simulink model "gm_max_frequency_index"  (R2020a)
settings: Solver=FixedStepDiscrete  StartTime=0.0  StopTime=1e-2  RelTol=1e-3
model workspace (MAT data in the model file):
  amplitud = 2047
  fft_length = 32
  samples_per_period = 3
  sampling_time = 1e-06
libraries: simulink x384, dspsrcs4 x1, dsphdlxfrm x1, dspstat3 x1, hdlsllib x1
(part 1 of 18)
settings Model: Creator=giova  LastModifiedBy=giova
settings SolverCC: AutoInsertRateTranBlk=on
settings DataIOCC: SaveOutput=off  SaveTime=off
settings OptimizationCC: BlockReduction=off  ConditionallyExecuteInputs=off  DefaultParameterBehavior=Inlined
settings DebuggingCC: AlgebraicLoopMsg=error  InheritedTsInSrcMsg=none  SingleTaskRateTransMsg=error  StrictBusMsg=ErrorOnBusTreatedAsVector  ArithmeticOperatorsInVariantConditions=warning
settings HardwareCC: ProdBitPerPointer=32  ProdBitPerSizeT=32  ProdBitPerPtrDiffT=32  ProdLargestAtomicFloat=None  ProdIntDivRoundTo=Undefined  ProdEndianess=Unspecified  ProdWordSize=32  ProdHWDeviceType=ASIC/FPGA->ASIC/FPGA  TargetBitPerPointer=64  TargetBitPerSizeT=64  TargetBitPerPtrDiffT=64  TargetLongLongMode=on  TargetIntDivRoundTo=Zero  TargetEndianess=LittleEndian  TargetWordSize=64  TargetHWDeviceType=Custom Processor->MATLAB Host Computer  ProdEqTarget=off
settings SFSimCC: SimUseLocalCustomCode=off  CustomCodeUndefinedFunction=UseInterfaceOnly
settings RTWCC: RTWUseLocalCustomCode=off
settings CodeAppCC: StateflowObjectComments=on
settings GRTTargetCC: TargetLangStandard=C89/C90 (ANSI)

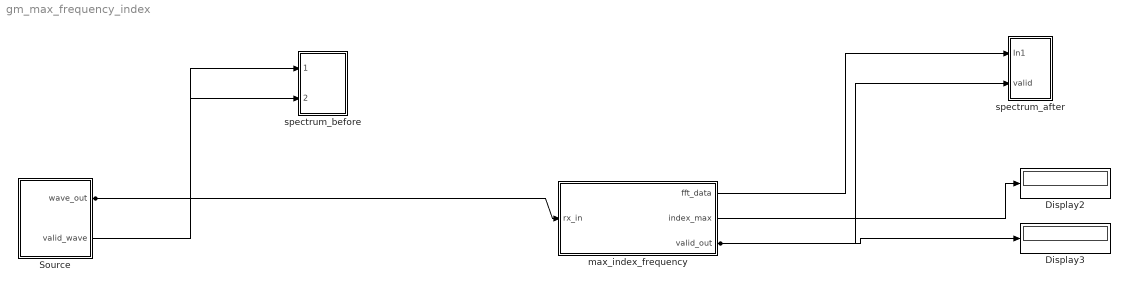
== system gm_max_frequency_index ==
  Display2 : Display
  Display3 : Display
  Source : Subsystem
  max_index_frequency : Subsystem
  spectrum_after : Subsystem
  spectrum_before : Subsystem
  wires:
  max_index_frequency/3(valid_out) -> Display3/1, spectrum_after/2(valid)
  max_index_frequency/2(index_max) -> Display2/1
  max_index_frequency/1(fft_data) -> spectrum_after/1(In1)
  Source/2(valid_wave) -> spectrum_before/2(valid_wave)
  Source/1(wave_out) -> max_index_frequency/1(rx_in), spectrum_before/1(wave_out)

== system gm_max_frequency_index/Source ==
  validated_wave : Subsystem
  wave_out : Outport  VectorParamsAs1DForOutWhenUnconnected=off
  valid_wave : Outport  Port=2  VectorParamsAs1DForOutWhenUnconnected=off
  wires:
  validated_wave/1(wave_out) -> wave_out/1
  validated_wave/2(valid) -> valid_wave/1

== system gm_max_frequency_index/max_index_frequency ==
  rx_in : Inport  OutDataTypeStr=fixdt(1, 12, 0)  PortDimensions=1  SampleTime=1e-06
      settings: SignalType=complex
  FFT_streamer : Subsystem
  frequency_max : Subsystem
  serial2parallel : Subsystem
  fft_data : Outport
  index_max : Outport  Port=2
  valid_out : Outport  Port=3
  wires:
  rx_in/1 -> serial2parallel/1(S)
  FFT_streamer/1(Out1) -> fft_data/1, frequency_max/1(fft_data)
  FFT_streamer/2(Out2) -> frequency_max/2(enable)
  frequency_max/1(index_max) -> index_max/1
  frequency_max/2(valid_out) -> valid_out/1
  serial2parallel/1(P) -> FFT_streamer/1(In1)
  serial2parallel/2(ValidOut) -> FFT_streamer/2(In2)

== system gm_max_frequency_index/spectrum_after ==
  In1 : Inport
  valid : Inport  Port=2
  Abs : Abs  OutDataTypeStr=single
  Cast To Single : DataTypeConversion  OutDataTypeStr=single
  Subsystem : Subsystem
  wires:
  valid/1 -> Subsystem/Enable
  Abs/1 -> Subsystem/1(In1)
  Cast To Single/1 -> Abs/1
  In1/1 -> Cast To Single/1

== system gm_max_frequency_index/spectrum_before ==
  wave_out : Inport
  valid_wave : Inport  Port=2
  Subsystem : Subsystem
  wires:
  valid_wave/1 -> Subsystem/Enable
  wave_out/1 -> Subsystem/1(In1)

== system gm_max_frequency_index/Source/validated_wave ==
  Start_pulse : Subsystem
  Wave_Generator : Subsystem
  wave_out : Outport  VectorParamsAs1DForOutWhenUnconnected=off
  valid : Outport  Port=2  VectorParamsAs1DForOutWhenUnconnected=off
  wires:
  Wave_Generator/1(wave_out) -> wave_out/1
  Start_pulse/1(Out1) -> Wave_Generator/Enable, valid/1

== system gm_max_frequency_index/max_index_frequency/FFT_streamer ==
  In1 : Inport  OutDataTypeStr=fixdt(1, 12, 0)  PortDimensions=[32]  SampleTime=3.2e-05
      settings: SignalType=complex
  In2 : Inport  Port=2  OutDataTypeStr=boolean  PortDimensions=1  SampleTime=3.2e-05
  FFT HDL Optimized : dsphdlxfrm/FFT HDL Optimized  FFTLength=fft_length  Architecture=Streaming Radix 2^2  ComplexMultiplication=Use 3 multipliers and 5 adders  BitReversedOutput=off  BitReversedInput=off  Normalize=on  SimulateUsing=Code generation  RoundingMethod=Floor  ResetInputPort=off  StartOutputPort=off  EndOutputPort=off
      settings: SourceProductBaseCode=DS
  Out1 : Outport
  Out2 : Outport  Port=2
  wires:
  FFT HDL Optimized/1 -> Out1/1
  FFT HDL Optimized/2 -> Out2/1
  In1/1 -> FFT HDL Optimized/1
  In2/1 -> FFT HDL Optimized/2

== system gm_max_frequency_index/max_index_frequency/frequency_max ==
  fft_data : Inport  OutDataTypeStr=fixdt(1, 12, 0)  PortDimensions=[32 1]  SampleTime=3.2e-05
      settings: SignalType=complex
  enable : Inport  Port=2  OutDataTypeStr=boolean  PortDimensions=1  SampleTime=3.2e-05
  index_finder : Subsystem
  index_max : Outport
  valid_out : Outport  Port=2
  wires:
  index_finder/1(index_max) -> index_max/1
  index_finder/2(valid_out) -> valid_out/1
  fft_data/1 -> index_finder/2(fft_data)
  enable/1 -> index_finder/1(enable)

== system gm_max_frequency_index/max_index_frequency/serial2parallel ==
  S : Inport  OutDataTypeStr=fixdt(1, 12, 0)  PortDimensions=1  SampleTime=1e-06
      settings: SignalType=complex
  Deserializer : hdlsllib/HDL Operations/Deserializer1D  Ratio=32  IdleCycles=0  InitialCondition="fi(0,1,12,0,\"hex\",\"000 + 000 i\")"  startIn=off  validIn=off  validOut=on  inputDataDimensions=1  inputSampleTime=1e-06  inputSignalType=complex
      settings: SourceProductBaseCode=SL
  P : Outport
  ValidOut : Outport  Port=2
  wires:
  Deserializer/1 -> P/1
  Deserializer/2 -> ValidOut/1
  S/1 -> Deserializer/1

== system gm_max_frequency_index/spectrum_after/Subsystem ==
  In1 : Inport
  Enable : EnablePort
  Spectrum Analyzer : SpectrumAnalyzer  IsFrequencyInputMode=1
  wires:
  In1/1 -> Spectrum Analyzer/1

== system gm_max_frequency_index/spectrum_before/Subsystem ==
  In1 : Inport
  Enable : EnablePort
  Spectrum Analyzer : SpectrumAnalyzer
  wires:
  In1/1 -> Spectrum Analyzer/1

== system gm_max_frequency_index/Source/validated_wave/Start_pulse ==
  Cast To Boolean : DataTypeConversion  OutDataTypeStr=boolean
  Constant : Constant  SampleTime=sampling_time  LockScale=on
  Out1 : Outport  VectorParamsAs1DForOutWhenUnconnected=off
  wires:
  Constant/1 -> Cast To Boolean/1
  Cast To Boolean/1 -> Out1/1

== system gm_max_frequency_index/Source/validated_wave/Wave_Generator ==
  enable_wave : EnablePort
  complex_wave : dspsrcs4/Sine Wave  Amplitude=amplitud  Frequency=1/(sampling_time*samples_per_period)  Phase=0  SampleMode=Discrete  OutComplex=Complex  CompMethod=Table lookup  TableSize=Speed  SampleTime=sampling_time  SamplesPerFrame=1  ResetState=Restart at time zero  OutputFrames=off  dataType=Fixed-point  wordLen=12  udDataType=sfix(16)  fracBitsMode=User-defined  numFracBits=0  OutDataTypeStr=fixdt(1,12,0)  LastOutDataTypeStr=fixdt(1,12,0)
  wave_out : Outport  InitialOutput=0  VectorParamsAs1DForOutWhenUnconnected=off
  wires:
  complex_wave/1 -> wave_out/1

== system gm_max_frequency_index/max_index_frequency/frequency_max/index_finder ==
  enable : Inport  OutDataTypeStr=boolean  PortDimensions=1  SampleTime=3.2e-05
  fft_data : Inport  Port=2  OutDataTypeStr=fixdt(1, 12, 0)  PortDimensions=[32 1]  SampleTime=3.2e-05
      settings: SignalType=complex
  Data Type Conversion : DataTypeConversion  OutDataTypeStr=uint8  SampleTime=3.2e-05
  Index Vector : MultiPortSwitch  DataPortOrder=Zero-based contiguous  Inputs=1  DiagnosticForDefault=None  zeroidx=on  SampleTime=3.2e-05
  Index Vector_dtc_comp : DataTypeConversion  OutDataTypeStr=fixdt(0, 5, 0)  SampleTime=3.2e-05  RndMeth=Zero
  Maximum : dspstat3/Maximum  operation=maximum  fcn=Index  indexBase=Zero  operateOver=Each column  Dimension=1  InputProcessing=Columns as channels (frame based)  reset=None  roiEnable=off  roiType=Rectangles  roiPortion=Entire ROI  roiOutput=Individual statistics for each ROI  roiFlag=off  roundingMode=Floor  overflowMode=off  prodOutputMode=Binary point scaling  prodOutputWordLength=16  prodOutputFracLength=0  prodOutputDataTypeStr=fixdt([],16,0)  prodOutputLastDataTypeStr=fixdt([],16,0)  accumMode=Binary point scaling  accumWordLength=16  accumFracLength=0  accumDataTypeStr=fixdt([],16,0)  accumLastDataTypeStr=fixdt([],16,0)
  for_each_instance1 : Subsystem
  for_each_instance10 : Subsystem
  for_each_instance11 : Subsystem
  for_each_instance12 : Subsystem
  for_each_instance13 : Subsystem
  for_each_instance14 : Subsystem
  for_each_instance15 : Subsystem
  for_each_instance16 : Subsystem
  for_each_instance17 : Subsystem
  for_each_instance18 : Subsystem
  for_each_instance19 : Subsystem
  for_each_instance2 : Subsystem
  for_each_instance20 : Subsystem
  for_each_instance21 : Subsystem
  for_each_instance22 : Subsystem
  for_each_instance23 : Subsystem
  for_each_instance24 : Subsystem
  for_each_instance25 : Subsystem
  for_each_instance26 : Subsystem
  for_each_instance27 : Subsystem
  for_each_instance28 : Subsystem
  for_each_instance29 : Subsystem
  for_each_instance3 : Subsystem
  for_each_instance30 : Subsystem
  for_each_instance31 : Subsystem
  for_each_instance32 : Subsystem
  for_each_instance4 : Subsystem
  for_each_instance5 : Subsystem
  for_each_instance6 : Subsystem
  for_each_instance7 : Subsystem
  for_each_instance8 : Subsystem
  for_each_instance9 : Subsystem
  t : Concatenate  NumInputs=32
  t1 : Reshape  OutputDimensionality=Column vector (2-D)
  t2 : Concatenate  NumInputs=32
  t3 : Reshape  OutputDimensionality=Column vector (2-D)
  t4 : Demux  Outputs=32
  index_max : Outport
  valid_out : Outport  Port=2
  wires:
  for_each_instance1/1(Out1) -> t2/1
  for_each_instance2/1(Out1) -> t2/2
  for_each_instance3/1(Out1) -> t2/3
  for_each_instance4/1(Out1) -> t2/4
  for_each_instance5/1(Out1) -> t2/5
  for_each_instance6/1(Out1) -> t2/6
  for_each_instance7/1(Out1) -> t2/7
  for_each_instance8/1(Out1) -> t2/8
  for_each_instance9/1(Out1) -> t2/9
  for_each_instance10/1(Out1) -> t2/10
  for_each_instance11/1(Out1) -> t2/11
  for_each_instance12/1(Out1) -> t2/12
  for_each_instance13/1(Out1) -> t2/13
  for_each_instance14/1(Out1) -> t2/14
  for_each_instance15/1(Out1) -> t2/15
  for_each_instance16/1(Out1) -> t2/16
  for_each_instance17/1(Out1) -> t2/17
  for_each_instance18/1(Out1) -> t2/18
  for_each_instance19/1(Out1) -> t2/19
  for_each_instance20/1(Out1) -> t2/20
  for_each_instance21/1(Out1) -> t2/21
  for_each_instance22/1(Out1) -> t2/22
  for_each_instance23/1(Out1) -> t2/23
  for_each_instance24/1(Out1) -> t2/24
  for_each_instance25/1(Out1) -> t2/25
  for_each_instance26/1(Out1) -> t2/26
  for_each_instance27/1(Out1) -> t2/27
  for_each_instance28/1(Out1) -> t2/28
  for_each_instance29/1(Out1) -> t2/29
  for_each_instance30/1(Out1) -> t2/30
  for_each_instance31/1(Out1) -> t2/31
  for_each_instance32/1(Out1) -> t2/32
  for_each_instance1/2(Out2) -> t/1
  for_each_instance2/2(Out2) -> t/2
  for_each_instance3/2(Out2) -> t/3
  for_each_instance4/2(Out2) -> t/4
  for_each_instance5/2(Out2) -> t/5
  for_each_instance6/2(Out2) -> t/6
  for_each_instance7/2(Out2) -> t/7
  for_each_instance8/2(Out2) -> t/8
  for_each_instance9/2(Out2) -> t/9
  for_each_instance10/2(Out2) -> t/10
  for_each_instance11/2(Out2) -> t/11
  for_each_instance12/2(Out2) -> t/12
  for_each_instance13/2(Out2) -> t/13
  for_each_instance14/2(Out2) -> t/14
  for_each_instance15/2(Out2) -> t/15
  for_each_instance16/2(Out2) -> t/16
  for_each_instance17/2(Out2) -> t/17
  for_each_instance18/2(Out2) -> t/18
  for_each_instance19/2(Out2) -> t/19
  for_each_instance20/2(Out2) -> t/20
  for_each_instance21/2(Out2) -> t/21
  for_each_instance22/2(Out2) -> t/22
  for_each_instance23/2(Out2) -> t/23
  for_each_instance24/2(Out2) -> t/24
  for_each_instance25/2(Out2) -> t/25
  for_each_instance26/2(Out2) -> t/26
  for_each_instance27/2(Out2) -> t/27
  for_each_instance28/2(Out2) -> t/28
  for_each_instance29/2(Out2) -> t/29
  for_each_instance30/2(Out2) -> t/30
  for_each_instance31/2(Out2) -> t/31
  for_each_instance32/2(Out2) -> t/32
  Data Type Conversion/1 -> index_max/1
  Index Vector/1 -> valid_out/1
  t4/1 -> for_each_instance1/1(fft_data)
  t4/2 -> for_each_instance2/1(fft_data)
  t4/3 -> for_each_instance3/1(fft_data)
  t4/4 -> for_each_instance4/1(fft_data)
  t4/5 -> for_each_instance5/1(fft_data)
  t4/6 -> for_each_instance6/1(fft_data)
  t4/7 -> for_each_instance7/1(fft_data)
  t4/8 -> for_each_instance8/1(fft_data)
  t4/9 -> for_each_instance9/1(fft_data)
  t4/10 -> for_each_instance10/1(fft_data)
  t4/11 -> for_each_instance11/1(fft_data)
  t4/12 -> for_each_instance12/1(fft_data)
  t4/13 -> for_each_instance13/1(fft_data)
  t4/14 -> for_each_instance14/1(fft_data)
  t4/15 -> for_each_instance15/1(fft_data)
  t4/16 -> for_each_instance16/1(fft_data)
  t4/17 -> for_each_instance17/1(fft_data)
  t4/18 -> for_each_instance18/1(fft_data)
  t4/19 -> for_each_instance19/1(fft_data)
  t4/20 -> for_each_instance20/1(fft_data)
  t4/21 -> for_each_instance21/1(fft_data)
  t4/22 -> for_each_instance22/1(fft_data)
  t4/23 -> for_each_instance23/1(fft_data)
  t4/24 -> for_each_instance24/1(fft_data)
  t4/25 -> for_each_instance25/1(fft_data)
  t4/26 -> for_each_instance26/1(fft_data)
  t4/27 -> for_each_instance27/1(fft_data)
  t4/28 -> for_each_instance28/1(fft_data)
  t4/29 -> for_each_instance29/1(fft_data)
  t4/30 -> for_each_instance30/1(fft_data)
  t4/31 -> for_each_instance31/1(fft_data)
  t4/32 -> for_each_instance32/1(fft_data)
  enable/1 -> for_each_instance32/2(enable), for_each_instance31/2(enable), for_each_instance30/2(enable), for_each_instance29/2(enable), for_each_instance28/2(enable), for_each_instance27/2(enable), for_each_instance26/2(enable), for_each_instance25/2(enable), for_each_instance24/2(enable), for_each_instance23/2(enable), for_each_instance22/2(enable), for_each_instance21/2(enable), for_each_instance20/2(enable), for_each_instance19/2(enable), for_each_instance18/2(enable), for_each_instance17/2(enable), for_each_instance16/2(enable), for_each_instance15/2(enable), for_each_instance14/2(enable), for_each_instance13/2(enable), for_each_instance12/2(enable), for_each_instance11/2(enable), for_each_instance10/2(enable), for_each_instance9/2(enable), for_each_instance8/2(enable), for_each_instance7/2(enable), for_each_instance6/2(enable), for_each_instance5/2(enable), for_each_instance4/2(enable), for_each_instance3/2(enable), for_each_instance2/2(enable), for_each_instance1/2(enable)
  fft_data/1 -> t4/1
  t/1 -> t1/1
  t1/1 -> Index Vector/2
  t2/1 -> t3/1
  t3/1 -> Maximum/1
  Maximum/1 -> Data Type Conversion/1, Index Vector_dtc_comp/1
  Index Vector_dtc_comp/1 -> Index Vector/1

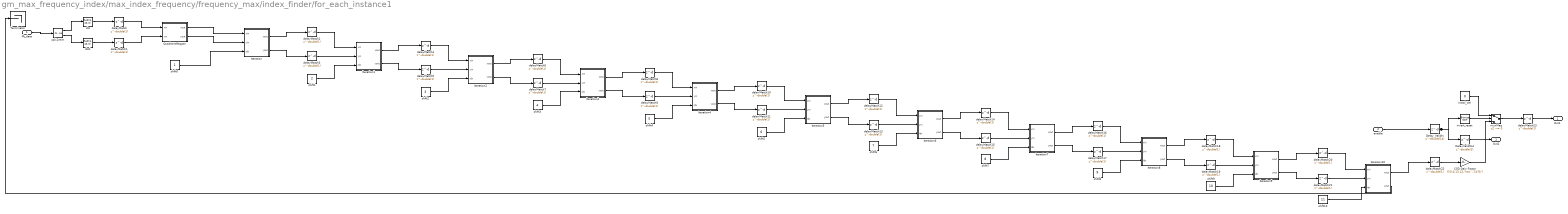
== system gm_max_frequency_index/max_index_frequency/frequency_max/index_finder/for_each_instance1 ==
  fft_data : Inport  OutDataTypeStr=fixdt(1, 12, 0)  PortDimensions=1  SampleTime=3.2e-05
      settings: SignalType=complex
  enable : Inport  Port=2  OutDataTypeStr=boolean  PortDimensions=1  SampleTime=3.2e-05
  CSD Gain Factor : Gain  Gain="fi(0,0,13,13,\"hex\",\"1b7b\")"  ParamDataTypeStr=fixdt(0, 13, 13)  OutDataTypeStr=fixdt(1, 13, 0)  SampleTime=3.2e-05
  DelayValidOut : Delay  DelayLength=double(1)  InitialCondition=0  SampleTime=3.2e-05
  Delay_ValidIn : Delay  DelayLength=double(14)  InitialCondition=0  SampleTime=3.2e-05
  Initial_Val : Constant  Value=0  OutDataTypeStr=fixdt(1, 13, 0)  SampleTime=3.2e-05
  Iteration : Subsystem
  Iteration1 : Subsystem
  Iteration10 : Subsystem
  Iteration2 : Subsystem
  Iteration3 : Subsystem
  Iteration4 : Subsystem
  Iteration5 : Subsystem
  Iteration6 : Subsystem
  Iteration7 : Subsystem
  Iteration8 : Subsystem
  Iteration9 : Subsystem
  QuadrantMapper : Subsystem
  Terminator : Terminator
  cplx2reim : ComplexToRealImag  SampleTime=3.2e-05
  delayMatch{,1..23} (24 alike) : Delay  DelayLength=double(1)  InitialCondition=0  SampleTime=3.2e-05
  dtc : DataTypeConversion  OutDataTypeStr=fixdt(1, 13, 0)  SampleTime=3.2e-05
  dtc1 : DataTypeConversion  OutDataTypeStr=fixdt(1, 13, 0)  SampleTime=3.2e-05
  invert_reset : simulink/Logic and Bit Operations/Bitwise Operator  logicop=NOT  UseBitMask=off  BitMask=double(0)  BitMaskRealWorld=Real World Value
  muxMag : Switch  Criteria=u2 ~= 0  Threshold=double(0)  OutDataTypeStr=fixdt(1, 13, 0)  SampleTime=3.2e-05
  shift0 : Constant  VectorParams1D=off  OutDataTypeStr=fixdt(0, 5, 0)  SampleTime=3.2e-05
  shift1 : Constant  Value=2  VectorParams1D=off  OutDataTypeStr=fixdt(0, 5, 0)  SampleTime=3.2e-05
  shift10 : Constant  Value=11  VectorParams1D=off  OutDataTypeStr=fixdt(0, 5, 0)  SampleTime=3.2e-05
  shift2 : Constant  Value=3  VectorParams1D=off  OutDataTypeStr=fixdt(0, 5, 0)  SampleTime=3.2e-05
  shift3 : Constant  Value=4  VectorParams1D=off  OutDataTypeStr=fixdt(0, 5, 0)  SampleTime=3.2e-05
  shift4 : Constant  Value=5  VectorParams1D=off  OutDataTypeStr=fixdt(0, 5, 0)  SampleTime=3.2e-05
  shift5 : Constant  Value=6  VectorParams1D=off  OutDataTypeStr=fixdt(0, 5, 0)  SampleTime=3.2e-05
  shift6 : Constant  Value=7  VectorParams1D=off  OutDataTypeStr=fixdt(0, 5, 0)  SampleTime=3.2e-05
  shift7 : Constant  Value=8  VectorParams1D=off  OutDataTypeStr=fixdt(0, 5, 0)  SampleTime=3.2e-05
  shift8 : Constant  Value=9  VectorParams1D=off  OutDataTypeStr=fixdt(0, 5, 0)  SampleTime=3.2e-05
  shift9 : Constant  Value=10  VectorParams1D=off  OutDataTypeStr=fixdt(0, 5, 0)  SampleTime=3.2e-05
  Out1 : Outport
  Out2 : Outport  Port=2  VectorParamsAs1DForOutWhenUnconnected=off
  wires:
  DelayValidOut/1 -> Out2/1
  delayMatch2/1 -> Iteration1/1(xin)
  delayMatch3/1 -> Iteration1/2(yin)
  delayMatch4/1 -> Iteration2/1(xin)
  delayMatch5/1 -> Iteration2/2(yin)
  delayMatch6/1 -> Iteration3/1(xin)
  delayMatch7/1 -> Iteration3/2(yin)
  delayMatch8/1 -> Iteration4/1(xin)
  delayMatch9/1 -> Iteration4/2(yin)
  delayMatch10/1 -> Iteration5/1(xin)
  delayMatch11/1 -> Iteration5/2(yin)
  delayMatch12/1 -> Iteration6/1(xin)
  delayMatch13/1 -> Iteration6/2(yin)
  delayMatch14/1 -> Iteration7/1(xin)
  delayMatch15/1 -> Iteration7/2(yin)
  delayMatch16/1 -> Iteration8/1(xin)
  delayMatch17/1 -> Iteration8/2(yin)
  delayMatch18/1 -> Iteration9/1(xin)
  delayMatch19/1 -> Iteration9/2(yin)
  delayMatch20/1 -> Iteration10/1(xin)
  delayMatch21/1 -> Iteration10/2(yin)
  delayMatch22/1 -> CSD Gain Factor/1
  delayMatch/1 -> QuadrantMapper/1(xin)
  delayMatch1/1 -> QuadrantMapper/2(yin)
  QuadrantMapper/1(xout) -> Iteration/1(xin)
  QuadrantMapper/2(yout) -> Iteration/2(yin)
  Delay_ValidIn/1 -> DelayValidOut/1, invert_reset/1
  delayMatch23/1 -> Out1/1
  fft_data/1 -> cplx2reim/1
  enable/1 -> Delay_ValidIn/1
  cplx2reim/1 -> dtc/1
  cplx2reim/2 -> dtc1/1
  dtc/1 -> delayMatch/1
  dtc1/1 -> delayMatch1/1
  shift0/1 -> Iteration/3(idx)
  Iteration/1(xout) -> delayMatch2/1
  Iteration/2(yout) -> delayMatch3/1
  shift1/1 -> Iteration1/3(idx)
  Iteration1/1(xout) -> delayMatch4/1
  Iteration1/2(yout) -> delayMatch5/1
  shift2/1 -> Iteration2/3(idx)
  Iteration2/1(xout) -> delayMatch6/1
  Iteration2/2(yout) -> delayMatch7/1
  shift3/1 -> Iteration3/3(idx)
  Iteration3/1(xout) -> delayMatch8/1
  Iteration3/2(yout) -> delayMatch9/1
  shift4/1 -> Iteration4/3(idx)
  Iteration4/1(xout) -> delayMatch10/1
  Iteration4/2(yout) -> delayMatch11/1
  shift5/1 -> Iteration5/3(idx)
  Iteration5/1(xout) -> delayMatch12/1
  Iteration5/2(yout) -> delayMatch13/1
  shift6/1 -> Iteration6/3(idx)
  Iteration6/1(xout) -> delayMatch14/1
  Iteration6/2(yout) -> delayMatch15/1
  shift7/1 -> Iteration7/3(idx)
  Iteration7/1(xout) -> delayMatch16/1
  Iteration7/2(yout) -> delayMatch17/1
  shift8/1 -> Iteration8/3(idx)
  Iteration8/1(xout) -> delayMatch18/1
  Iteration8/2(yout) -> delayMatch19/1
  shift9/1 -> Iteration9/3(idx)
  Iteration9/1(xout) -> delayMatch20/1
  Iteration9/2(yout) -> delayMatch21/1
  Iteration10/2(yout) -> Terminator/1
  shift10/1 -> Iteration10/3(idx)
  Iteration10/1(xout) -> delayMatch22/1
  Initial_Val/1 -> muxMag/1
  CSD Gain Factor/1 -> muxMag/3
  invert_reset/1 -> muxMag/2
  muxMag/1 -> delayMatch23/1

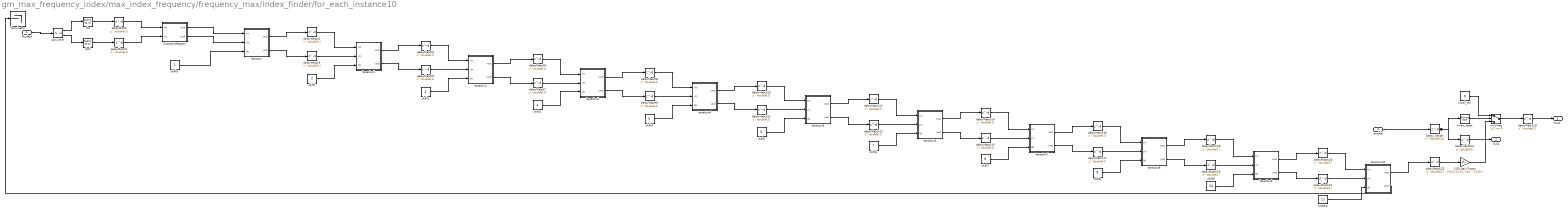
== system gm_max_frequency_index/max_index_frequency/frequency_max/index_finder/for_each_instance10 ==
  fft_data : Inport  OutDataTypeStr=fixdt(1, 12, 0)  PortDimensions=1  SampleTime=3.2e-05
      settings: SignalType=complex
  enable : Inport  Port=2  OutDataTypeStr=boolean  PortDimensions=1  SampleTime=3.2e-05
  CSD Gain Factor : Gain  Gain="fi(0,0,13,13,\"hex\",\"1b7b\")"  ParamDataTypeStr=fixdt(0, 13, 13)  OutDataTypeStr=fixdt(1, 13, 0)  SampleTime=3.2e-05
  DelayValidOut : Delay  DelayLength=double(1)  InitialCondition=0  SampleTime=3.2e-05
  Delay_ValidIn : Delay  DelayLength=double(14)  InitialCondition=0  SampleTime=3.2e-05
  Initial_Val : Constant  Value=0  OutDataTypeStr=fixdt(1, 13, 0)  SampleTime=3.2e-05
  Iteration : Subsystem
  Iteration1 : Subsystem
  Iteration10 : Subsystem
  Iteration2 : Subsystem
  Iteration3 : Subsystem
  Iteration4 : Subsystem
  Iteration5 : Subsystem
  Iteration6 : Subsystem
  Iteration7 : Subsystem
  Iteration8 : Subsystem
  Iteration9 : Subsystem
  QuadrantMapper : Subsystem
  Terminator : Terminator
  cplx2reim : ComplexToRealImag  SampleTime=3.2e-05
  delayMatch{,1..23} (24 alike) : Delay  DelayLength=double(1)  InitialCondition=0  SampleTime=3.2e-05
  dtc : DataTypeConversion  OutDataTypeStr=fixdt(1, 13, 0)  SampleTime=3.2e-05
  dtc1 : DataTypeConversion  OutDataTypeStr=fixdt(1, 13, 0)  SampleTime=3.2e-05
  invert_reset : simulink/Logic and Bit Operations/Bitwise Operator  logicop=NOT  UseBitMask=off  BitMask=double(0)  BitMaskRealWorld=Real World Value
  muxMag : Switch  Criteria=u2 ~= 0  Threshold=double(0)  OutDataTypeStr=fixdt(1, 13, 0)  SampleTime=3.2e-05
  shift0 : Constant  VectorParams1D=off  OutDataTypeStr=fixdt(0, 5, 0)  SampleTime=3.2e-05
  shift1 : Constant  Value=2  VectorParams1D=off  OutDataTypeStr=fixdt(0, 5, 0)  SampleTime=3.2e-05
  shift10 : Constant  Value=11  VectorParams1D=off  OutDataTypeStr=fixdt(0, 5, 0)  SampleTime=3.2e-05
  shift2 : Constant  Value=3  VectorParams1D=off  OutDataTypeStr=fixdt(0, 5, 0)  SampleTime=3.2e-05
  shift3 : Constant  Value=4  VectorParams1D=off  OutDataTypeStr=fixdt(0, 5, 0)  SampleTime=3.2e-05
  shift4 : Constant  Value=5  VectorParams1D=off  OutDataTypeStr=fixdt(0, 5, 0)  SampleTime=3.2e-05
  shift5 : Constant  Value=6  VectorParams1D=off  OutDataTypeStr=fixdt(0, 5, 0)  SampleTime=3.2e-05
  shift6 : Constant  Value=7  VectorParams1D=off  OutDataTypeStr=fixdt(0, 5, 0)  SampleTime=3.2e-05
  shift7 : Constant  Value=8  VectorParams1D=off  OutDataTypeStr=fixdt(0, 5, 0)  SampleTime=3.2e-05
  shift8 : Constant  Value=9  VectorParams1D=off  OutDataTypeStr=fixdt(0, 5, 0)  SampleTime=3.2e-05
  shift9 : Constant  Value=10  VectorParams1D=off  OutDataTypeStr=fixdt(0, 5, 0)  SampleTime=3.2e-05
  Out1 : Outport
  Out2 : Outport  Port=2  VectorParamsAs1DForOutWhenUnconnected=off
  wires:
  muxMag/1 -> delayMatch23/1
  invert_reset/1 -> muxMag/2
  CSD Gain Factor/1 -> muxMag/3
  Initial_Val/1 -> muxMag/1
  Iteration10/1(xout) -> delayMatch22/1
  shift10/1 -> Iteration10/3(idx)
  Iteration10/2(yout) -> Terminator/1
  Iteration9/2(yout) -> delayMatch21/1
  Iteration9/1(xout) -> delayMatch20/1
  shift9/1 -> Iteration9/3(idx)
  Iteration8/2(yout) -> delayMatch19/1
  Iteration8/1(xout) -> delayMatch18/1
  shift8/1 -> Iteration8/3(idx)
  Iteration7/2(yout) -> delayMatch17/1
  Iteration7/1(xout) -> delayMatch16/1
  shift7/1 -> Iteration7/3(idx)
  Iteration6/2(yout) -> delayMatch15/1
  Iteration6/1(xout) -> delayMatch14/1
  shift6/1 -> Iteration6/3(idx)
  Iteration5/2(yout) -> delayMatch13/1
  Iteration5/1(xout) -> delayMatch12/1
  shift5/1 -> Iteration5/3(idx)
  Iteration4/2(yout) -> delayMatch11/1
  Iteration4/1(xout) -> delayMatch10/1
  shift4/1 -> Iteration4/3(idx)
  Iteration3/2(yout) -> delayMatch9/1
  Iteration3/1(xout) -> delayMatch8/1
  shift3/1 -> Iteration3/3(idx)
  Iteration2/2(yout) -> delayMatch7/1
  Iteration2/1(xout) -> delayMatch6/1
  shift2/1 -> Iteration2/3(idx)
  Iteration1/2(yout) -> delayMatch5/1
  Iteration1/1(xout) -> delayMatch4/1
  shift1/1 -> Iteration1/3(idx)
  Iteration/2(yout) -> delayMatch3/1
  Iteration/1(xout) -> delayMatch2/1
  shift0/1 -> Iteration/3(idx)
  dtc1/1 -> delayMatch1/1
  dtc/1 -> delayMatch/1
  cplx2reim/2 -> dtc1/1
  cplx2reim/1 -> dtc/1
  enable/1 -> Delay_ValidIn/1
  fft_data/1 -> cplx2reim/1
  delayMatch23/1 -> Out1/1
  Delay_ValidIn/1 -> invert_reset/1, DelayValidOut/1
  QuadrantMapper/2(yout) -> Iteration/2(yin)
  QuadrantMapper/1(xout) -> Iteration/1(xin)
  delayMatch1/1 -> QuadrantMapper/2(yin)
  delayMatch/1 -> QuadrantMapper/1(xin)
  delayMatch22/1 -> CSD Gain Factor/1
  delayMatch21/1 -> Iteration10/2(yin)
  delayMatch20/1 -> Iteration10/1(xin)
  delayMatch19/1 -> Iteration9/2(yin)
  delayMatch18/1 -> Iteration9/1(xin)
  delayMatch17/1 -> Iteration8/2(yin)
  delayMatch16/1 -> Iteration8/1(xin)
  delayMatch15/1 -> Iteration7/2(yin)
  delayMatch14/1 -> Iteration7/1(xin)
  delayMatch13/1 -> Iteration6/2(yin)
  delayMatch12/1 -> Iteration6/1(xin)
  delayMatch11/1 -> Iteration5/2(yin)
  delayMatch10/1 -> Iteration5/1(xin)
  delayMatch9/1 -> Iteration4/2(yin)
  delayMatch8/1 -> Iteration4/1(xin)
  delayMatch7/1 -> Iteration3/2(yin)
  delayMatch6/1 -> Iteration3/1(xin)
  delayMatch5/1 -> Iteration2/2(yin)
  delayMatch4/1 -> Iteration2/1(xin)
  delayMatch3/1 -> Iteration1/2(yin)
  delayMatch2/1 -> Iteration1/1(xin)
  DelayValidOut/1 -> Out2/1

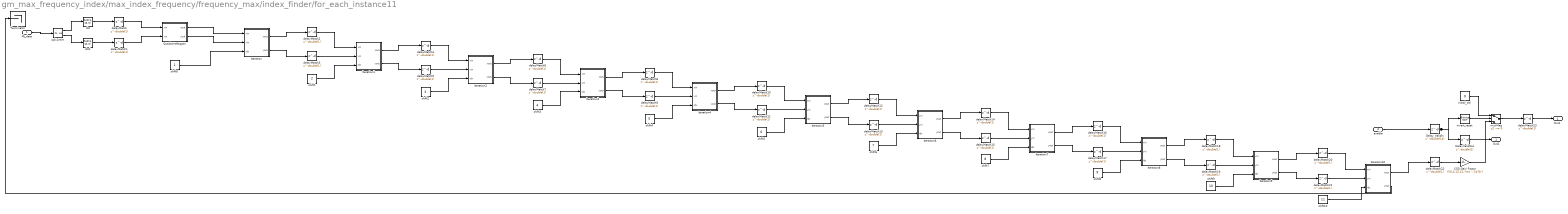
== system gm_max_frequency_index/max_index_frequency/frequency_max/index_finder/for_each_instance11 ==
  fft_data : Inport  OutDataTypeStr=fixdt(1, 12, 0)  PortDimensions=1  SampleTime=3.2e-05
      settings: SignalType=complex
  enable : Inport  Port=2  OutDataTypeStr=boolean  PortDimensions=1  SampleTime=3.2e-05
  CSD Gain Factor : Gain  Gain="fi(0,0,13,13,\"hex\",\"1b7b\")"  ParamDataTypeStr=fixdt(0, 13, 13)  OutDataTypeStr=fixdt(1, 13, 0)  SampleTime=3.2e-05
  DelayValidOut : Delay  DelayLength=double(1)  InitialCondition=0  SampleTime=3.2e-05
  Delay_ValidIn : Delay  DelayLength=double(14)  InitialCondition=0  SampleTime=3.2e-05
  Initial_Val : Constant  Value=0  OutDataTypeStr=fixdt(1, 13, 0)  SampleTime=3.2e-05
  Iteration : Subsystem
  Iteration1 : Subsystem
  Iteration10 : Subsystem
  Iteration2 : Subsystem
  Iteration3 : Subsystem
  Iteration4 : Subsystem
  Iteration5 : Subsystem
  Iteration6 : Subsystem
  Iteration7 : Subsystem
  Iteration8 : Subsystem
  Iteration9 : Subsystem
  QuadrantMapper : Subsystem
  Terminator : Terminator
  cplx2reim : ComplexToRealImag  SampleTime=3.2e-05
  delayMatch{,1..23} (24 alike) : Delay  DelayLength=double(1)  InitialCondition=0  SampleTime=3.2e-05
  dtc : DataTypeConversion  OutDataTypeStr=fixdt(1, 13, 0)  SampleTime=3.2e-05
  dtc1 : DataTypeConversion  OutDataTypeStr=fixdt(1, 13, 0)  SampleTime=3.2e-05
  invert_reset : simulink/Logic and Bit Operations/Bitwise Operator  logicop=NOT  UseBitMask=off  BitMask=double(0)  BitMaskRealWorld=Real World Value
  muxMag : Switch  Criteria=u2 ~= 0  Threshold=double(0)  OutDataTypeStr=fixdt(1, 13, 0)  SampleTime=3.2e-05
  shift0 : Constant  VectorParams1D=off  OutDataTypeStr=fixdt(0, 5, 0)  SampleTime=3.2e-05
  shift1 : Constant  Value=2  VectorParams1D=off  OutDataTypeStr=fixdt(0, 5, 0)  SampleTime=3.2e-05
  shift10 : Constant  Value=11  VectorParams1D=off  OutDataTypeStr=fixdt(0, 5, 0)  SampleTime=3.2e-05
  shift2 : Constant  Value=3  VectorParams1D=off  OutDataTypeStr=fixdt(0, 5, 0)  SampleTime=3.2e-05
  shift3 : Constant  Value=4  VectorParams1D=off  OutDataTypeStr=fixdt(0, 5, 0)  SampleTime=3.2e-05
  shift4 : Constant  Value=5  VectorParams1D=off  OutDataTypeStr=fixdt(0, 5, 0)  SampleTime=3.2e-05
  shift5 : Constant  Value=6  VectorParams1D=off  OutDataTypeStr=fixdt(0, 5, 0)  SampleTime=3.2e-05
  shift6 : Constant  Value=7  VectorParams1D=off  OutDataTypeStr=fixdt(0, 5, 0)  SampleTime=3.2e-05
  shift7 : Constant  Value=8  VectorParams1D=off  OutDataTypeStr=fixdt(0, 5, 0)  SampleTime=3.2e-05
  shift8 : Constant  Value=9  VectorParams1D=off  OutDataTypeStr=fixdt(0, 5, 0)  SampleTime=3.2e-05
  shift9 : Constant  Value=10  VectorParams1D=off  OutDataTypeStr=fixdt(0, 5, 0)  SampleTime=3.2e-05
  Out1 : Outport
  Out2 : Outport  Port=2  VectorParamsAs1DForOutWhenUnconnected=off
  wires:
  muxMag/1 -> delayMatch23/1
  invert_reset/1 -> muxMag/2
  CSD Gain Factor/1 -> muxMag/3
  Initial_Val/1 -> muxMag/1
  Iteration10/1(xout) -> delayMatch22/1
  shift10/1 -> Iteration10/3(idx)
  Iteration10/2(yout) -> Terminator/1
  Iteration9/2(yout) -> delayMatch21/1
  Iteration9/1(xout) -> delayMatch20/1
  shift9/1 -> Iteration9/3(idx)
  Iteration8/2(yout) -> delayMatch19/1
  Iteration8/1(xout) -> delayMatch18/1
  shift8/1 -> Iteration8/3(idx)
  Iteration7/2(yout) -> delayMatch17/1
  Iteration7/1(xout) -> delayMatch16/1
  shift7/1 -> Iteration7/3(idx)
  Iteration6/2(yout) -> delayMatch15/1
  Iteration6/1(xout) -> delayMatch14/1
  shift6/1 -> Iteration6/3(idx)
  Iteration5/2(yout) -> delayMatch13/1
  Iteration5/1(xout) -> delayMatch12/1
  shift5/1 -> Iteration5/3(idx)
  Iteration4/2(yout) -> delayMatch11/1
  Iteration4/1(xout) -> delayMatch10/1
  shift4/1 -> Iteration4/3(idx)
  Iteration3/2(yout) -> delayMatch9/1
  Iteration3/1(xout) -> delayMatch8/1
  shift3/1 -> Iteration3/3(idx)
  Iteration2/2(yout) -> delayMatch7/1
  Iteration2/1(xout) -> delayMatch6/1
  shift2/1 -> Iteration2/3(idx)
  Iteration1/2(yout) -> delayMatch5/1
  Iteration1/1(xout) -> delayMatch4/1
  shift1/1 -> Iteration1/3(idx)
  Iteration/2(yout) -> delayMatch3/1
  Iteration/1(xout) -> delayMatch2/1
  shift0/1 -> Iteration/3(idx)
  dtc1/1 -> delayMatch1/1
  dtc/1 -> delayMatch/1
  cplx2reim/2 -> dtc1/1
  cplx2reim/1 -> dtc/1
  enable/1 -> Delay_ValidIn/1
  fft_data/1 -> cplx2reim/1
  delayMatch23/1 -> Out1/1
  Delay_ValidIn/1 -> invert_reset/1, DelayValidOut/1
  QuadrantMapper/2(yout) -> Iteration/2(yin)
  QuadrantMapper/1(xout) -> Iteration/1(xin)
  delayMatch1/1 -> QuadrantMapper/2(yin)
  delayMatch/1 -> QuadrantMapper/1(xin)
  delayMatch22/1 -> CSD Gain Factor/1
  delayMatch21/1 -> Iteration10/2(yin)
  delayMatch20/1 -> Iteration10/1(xin)
  delayMatch19/1 -> Iteration9/2(yin)
  delayMatch18/1 -> Iteration9/1(xin)
  delayMatch17/1 -> Iteration8/2(yin)
  delayMatch16/1 -> Iteration8/1(xin)
  delayMatch15/1 -> Iteration7/2(yin)
  delayMatch14/1 -> Iteration7/1(xin)
  delayMatch13/1 -> Iteration6/2(yin)
  delayMatch12/1 -> Iteration6/1(xin)
  delayMatch11/1 -> Iteration5/2(yin)
  delayMatch10/1 -> Iteration5/1(xin)
  delayMatch9/1 -> Iteration4/2(yin)
  delayMatch8/1 -> Iteration4/1(xin)
  delayMatch7/1 -> Iteration3/2(yin)
  delayMatch6/1 -> Iteration3/1(xin)
  delayMatch5/1 -> Iteration2/2(yin)
  delayMatch4/1 -> Iteration2/1(xin)
  delayMatch3/1 -> Iteration1/2(yin)
  delayMatch2/1 -> Iteration1/1(xin)
  DelayValidOut/1 -> Out2/1

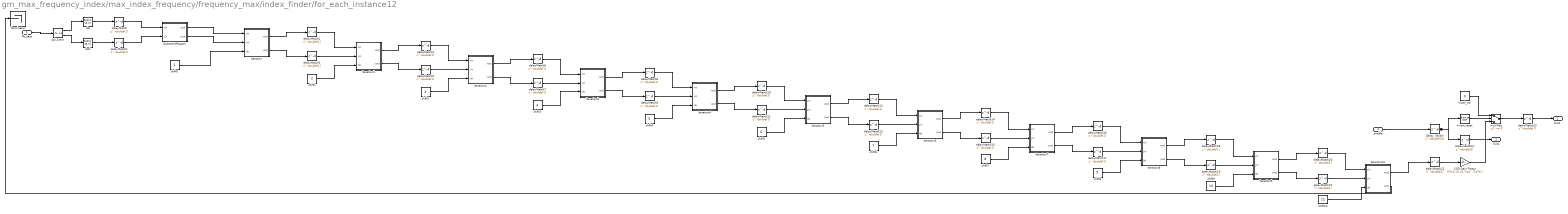
== system gm_max_frequency_index/max_index_frequency/frequency_max/index_finder/for_each_instance12 ==
  fft_data : Inport  OutDataTypeStr=fixdt(1, 12, 0)  PortDimensions=1  SampleTime=3.2e-05
      settings: SignalType=complex
  enable : Inport  Port=2  OutDataTypeStr=boolean  PortDimensions=1  SampleTime=3.2e-05
  CSD Gain Factor : Gain  Gain="fi(0,0,13,13,\"hex\",\"1b7b\")"  ParamDataTypeStr=fixdt(0, 13, 13)  OutDataTypeStr=fixdt(1, 13, 0)  SampleTime=3.2e-05
  DelayValidOut : Delay  DelayLength=double(1)  InitialCondition=0  SampleTime=3.2e-05
  Delay_ValidIn : Delay  DelayLength=double(14)  InitialCondition=0  SampleTime=3.2e-05
  Initial_Val : Constant  Value=0  OutDataTypeStr=fixdt(1, 13, 0)  SampleTime=3.2e-05
  Iteration : Subsystem
  Iteration1 : Subsystem
  Iteration10 : Subsystem
  Iteration2 : Subsystem
  Iteration3 : Subsystem
  Iteration4 : Subsystem
  Iteration5 : Subsystem
  Iteration6 : Subsystem
  Iteration7 : Subsystem
  Iteration8 : Subsystem
  Iteration9 : Subsystem
  QuadrantMapper : Subsystem
  Terminator : Terminator
  cplx2reim : ComplexToRealImag  SampleTime=3.2e-05
  delayMatch{,1..23} (24 alike) : Delay  DelayLength=double(1)  InitialCondition=0  SampleTime=3.2e-05
  dtc : DataTypeConversion  OutDataTypeStr=fixdt(1, 13, 0)  SampleTime=3.2e-05
  dtc1 : DataTypeConversion  OutDataTypeStr=fixdt(1, 13, 0)  SampleTime=3.2e-05
  invert_reset : simulink/Logic and Bit Operations/Bitwise Operator  logicop=NOT  UseBitMask=off  BitMask=double(0)  BitMaskRealWorld=Real World Value
  muxMag : Switch  Criteria=u2 ~= 0  Threshold=double(0)  OutDataTypeStr=fixdt(1, 13, 0)  SampleTime=3.2e-05
  shift0 : Constant  VectorParams1D=off  OutDataTypeStr=fixdt(0, 5, 0)  SampleTime=3.2e-05
  shift1 : Constant  Value=2  VectorParams1D=off  OutDataTypeStr=fixdt(0, 5, 0)  SampleTime=3.2e-05
  shift10 : Constant  Value=11  VectorParams1D=off  OutDataTypeStr=fixdt(0, 5, 0)  SampleTime=3.2e-05
  shift2 : Constant  Value=3  VectorParams1D=off  OutDataTypeStr=fixdt(0, 5, 0)  SampleTime=3.2e-05
  shift3 : Constant  Value=4  VectorParams1D=off  OutDataTypeStr=fixdt(0, 5, 0)  SampleTime=3.2e-05
  shift4 : Constant  Value=5  VectorParams1D=off  OutDataTypeStr=fixdt(0, 5, 0)  SampleTime=3.2e-05
  shift5 : Constant  Value=6  VectorParams1D=off  OutDataTypeStr=fixdt(0, 5, 0)  SampleTime=3.2e-05
  shift6 : Constant  Value=7  VectorParams1D=off  OutDataTypeStr=fixdt(0, 5, 0)  SampleTime=3.2e-05
  shift7 : Constant  Value=8  VectorParams1D=off  OutDataTypeStr=fixdt(0, 5, 0)  SampleTime=3.2e-05
  shift8 : Constant  Value=9  VectorParams1D=off  OutDataTypeStr=fixdt(0, 5, 0)  SampleTime=3.2e-05
  shift9 : Constant  Value=10  VectorParams1D=off  OutDataTypeStr=fixdt(0, 5, 0)  SampleTime=3.2e-05
  Out1 : Outport
  Out2 : Outport  Port=2  VectorParamsAs1DForOutWhenUnconnected=off
  wires:
  muxMag/1 -> delayMatch23/1
  invert_reset/1 -> muxMag/2
  CSD Gain Factor/1 -> muxMag/3
  Initial_Val/1 -> muxMag/1
  Iteration10/1(xout) -> delayMatch22/1
  shift10/1 -> Iteration10/3(idx)
  Iteration10/2(yout) -> Terminator/1
  Iteration9/2(yout) -> delayMatch21/1
  Iteration9/1(xout) -> delayMatch20/1
  shift9/1 -> Iteration9/3(idx)
  Iteration8/2(yout) -> delayMatch19/1
  Iteration8/1(xout) -> delayMatch18/1
  shift8/1 -> Iteration8/3(idx)
  Iteration7/2(yout) -> delayMatch17/1
  Iteration7/1(xout) -> delayMatch16/1
  shift7/1 -> Iteration7/3(idx)
  Iteration6/2(yout) -> delayMatch15/1
  Iteration6/1(xout) -> delayMatch14/1
  shift6/1 -> Iteration6/3(idx)
  Iteration5/2(yout) -> delayMatch13/1
  Iteration5/1(xout) -> delayMatch12/1
  shift5/1 -> Iteration5/3(idx)
  Iteration4/2(yout) -> delayMatch11/1
  Iteration4/1(xout) -> delayMatch10/1
  shift4/1 -> Iteration4/3(idx)
  Iteration3/2(yout) -> delayMatch9/1
  Iteration3/1(xout) -> delayMatch8/1
  shift3/1 -> Iteration3/3(idx)
  Iteration2/2(yout) -> delayMatch7/1
  Iteration2/1(xout) -> delayMatch6/1
  shift2/1 -> Iteration2/3(idx)
  Iteration1/2(yout) -> delayMatch5/1
  Iteration1/1(xout) -> delayMatch4/1
  shift1/1 -> Iteration1/3(idx)
  Iteration/2(yout) -> delayMatch3/1
  Iteration/1(xout) -> delayMatch2/1
  shift0/1 -> Iteration/3(idx)
  dtc1/1 -> delayMatch1/1
  dtc/1 -> delayMatch/1
  cplx2reim/2 -> dtc1/1
  cplx2reim/1 -> dtc/1
  enable/1 -> Delay_ValidIn/1
  fft_data/1 -> cplx2reim/1
  delayMatch23/1 -> Out1/1
  Delay_ValidIn/1 -> invert_reset/1, DelayValidOut/1
  QuadrantMapper/2(yout) -> Iteration/2(yin)
  QuadrantMapper/1(xout) -> Iteration/1(xin)
  delayMatch1/1 -> QuadrantMapper/2(yin)
  delayMatch/1 -> QuadrantMapper/1(xin)
  delayMatch22/1 -> CSD Gain Factor/1
  delayMatch21/1 -> Iteration10/2(yin)
  delayMatch20/1 -> Iteration10/1(xin)
  delayMatch19/1 -> Iteration9/2(yin)
  delayMatch18/1 -> Iteration9/1(xin)
  delayMatch17/1 -> Iteration8/2(yin)
  delayMatch16/1 -> Iteration8/1(xin)
  delayMatch15/1 -> Iteration7/2(yin)
  delayMatch14/1 -> Iteration7/1(xin)
  delayMatch13/1 -> Iteration6/2(yin)
  delayMatch12/1 -> Iteration6/1(xin)
  delayMatch11/1 -> Iteration5/2(yin)
  delayMatch10/1 -> Iteration5/1(xin)
  delayMatch9/1 -> Iteration4/2(yin)
  delayMatch8/1 -> Iteration4/1(xin)
  delayMatch7/1 -> Iteration3/2(yin)
  delayMatch6/1 -> Iteration3/1(xin)
  delayMatch5/1 -> Iteration2/2(yin)
  delayMatch4/1 -> Iteration2/1(xin)
  delayMatch3/1 -> Iteration1/2(yin)
  delayMatch2/1 -> Iteration1/1(xin)
  DelayValidOut/1 -> Out2/1

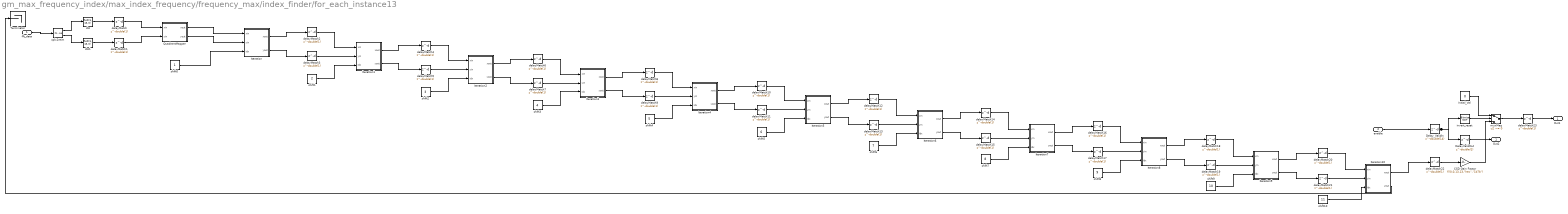
== system gm_max_frequency_index/max_index_frequency/frequency_max/index_finder/for_each_instance13 ==
  fft_data : Inport  OutDataTypeStr=fixdt(1, 12, 0)  PortDimensions=1  SampleTime=3.2e-05
      settings: SignalType=complex
  enable : Inport  Port=2  OutDataTypeStr=boolean  PortDimensions=1  SampleTime=3.2e-05
  CSD Gain Factor : Gain  Gain="fi(0,0,13,13,\"hex\",\"1b7b\")"  ParamDataTypeStr=fixdt(0, 13, 13)  OutDataTypeStr=fixdt(1, 13, 0)  SampleTime=3.2e-05
  DelayValidOut : Delay  DelayLength=double(1)  InitialCondition=0  SampleTime=3.2e-05
  Delay_ValidIn : Delay  DelayLength=double(14)  InitialCondition=0  SampleTime=3.2e-05
  Initial_Val : Constant  Value=0  OutDataTypeStr=fixdt(1, 13, 0)  SampleTime=3.2e-05
  Iteration : Subsystem
  Iteration1 : Subsystem
  Iteration10 : Subsystem
  Iteration2 : Subsystem
  Iteration3 : Subsystem
  Iteration4 : Subsystem
  Iteration5 : Subsystem
  Iteration6 : Subsystem
  Iteration7 : Subsystem
  Iteration8 : Subsystem
  Iteration9 : Subsystem
  QuadrantMapper : Subsystem
  Terminator : Terminator
  cplx2reim : ComplexToRealImag  SampleTime=3.2e-05
  delayMatch{,1..23} (24 alike) : Delay  DelayLength=double(1)  InitialCondition=0  SampleTime=3.2e-05
  dtc : DataTypeConversion  OutDataTypeStr=fixdt(1, 13, 0)  SampleTime=3.2e-05
  dtc1 : DataTypeConversion  OutDataTypeStr=fixdt(1, 13, 0)  SampleTime=3.2e-05
  invert_reset : simulink/Logic and Bit Operations/Bitwise Operator  logicop=NOT  UseBitMask=off  BitMask=double(0)  BitMaskRealWorld=Real World Value
  muxMag : Switch  Criteria=u2 ~= 0  Threshold=double(0)  OutDataTypeStr=fixdt(1, 13, 0)  SampleTime=3.2e-05
  shift0 : Constant  VectorParams1D=off  OutDataTypeStr=fixdt(0, 5, 0)  SampleTime=3.2e-05
  shift1 : Constant  Value=2  VectorParams1D=off  OutDataTypeStr=fixdt(0, 5, 0)  SampleTime=3.2e-05
  shift10 : Constant  Value=11  VectorParams1D=off  OutDataTypeStr=fixdt(0, 5, 0)  SampleTime=3.2e-05
  shift2 : Constant  Value=3  VectorParams1D=off  OutDataTypeStr=fixdt(0, 5, 0)  SampleTime=3.2e-05
  shift3 : Constant  Value=4  VectorParams1D=off  OutDataTypeStr=fixdt(0, 5, 0)  SampleTime=3.2e-05
  shift4 : Constant  Value=5  VectorParams1D=off  OutDataTypeStr=fixdt(0, 5, 0)  SampleTime=3.2e-05
  shift5 : Constant  Value=6  VectorParams1D=off  OutDataTypeStr=fixdt(0, 5, 0)  SampleTime=3.2e-05
  shift6 : Constant  Value=7  VectorParams1D=off  OutDataTypeStr=fixdt(0, 5, 0)  SampleTime=3.2e-05
  shift7 : Constant  Value=8  VectorParams1D=off  OutDataTypeStr=fixdt(0, 5, 0)  SampleTime=3.2e-05
  shift8 : Constant  Value=9  VectorParams1D=off  OutDataTypeStr=fixdt(0, 5, 0)  SampleTime=3.2e-05
  shift9 : Constant  Value=10  VectorParams1D=off  OutDataTypeStr=fixdt(0, 5, 0)  SampleTime=3.2e-05
  Out1 : Outport
  Out2 : Outport  Port=2  VectorParamsAs1DForOutWhenUnconnected=off
  wires:
  muxMag/1 -> delayMatch23/1
  invert_reset/1 -> muxMag/2
  CSD Gain Factor/1 -> muxMag/3
  Initial_Val/1 -> muxMag/1
  Iteration10/1(xout) -> delayMatch22/1
  shift10/1 -> Iteration10/3(idx)
  Iteration10/2(yout) -> Terminator/1
  Iteration9/2(yout) -> delayMatch21/1
  Iteration9/1(xout) -> delayMatch20/1
  shift9/1 -> Iteration9/3(idx)
  Iteration8/2(yout) -> delayMatch19/1
  Iteration8/1(xout) -> delayMatch18/1
  shift8/1 -> Iteration8/3(idx)
  Iteration7/2(yout) -> delayMatch17/1
  Iteration7/1(xout) -> delayMatch16/1
  shift7/1 -> Iteration7/3(idx)
  Iteration6/2(yout) -> delayMatch15/1
  Iteration6/1(xout) -> delayMatch14/1
  shift6/1 -> Iteration6/3(idx)
  Iteration5/2(yout) -> delayMatch13/1
  Iteration5/1(xout) -> delayMatch12/1
  shift5/1 -> Iteration5/3(idx)
  Iteration4/2(yout) -> delayMatch11/1
  Iteration4/1(xout) -> delayMatch10/1
  shift4/1 -> Iteration4/3(idx)
  Iteration3/2(yout) -> delayMatch9/1
  Iteration3/1(xout) -> delayMatch8/1
  shift3/1 -> Iteration3/3(idx)
  Iteration2/2(yout) -> delayMatch7/1
  Iteration2/1(xout) -> delayMatch6/1
  shift2/1 -> Iteration2/3(idx)
  Iteration1/2(yout) -> delayMatch5/1
  Iteration1/1(xout) -> delayMatch4/1
  shift1/1 -> Iteration1/3(idx)
  Iteration/2(yout) -> delayMatch3/1
  Iteration/1(xout) -> delayMatch2/1
  shift0/1 -> Iteration/3(idx)
  dtc1/1 -> delayMatch1/1
  dtc/1 -> delayMatch/1
  cplx2reim/2 -> dtc1/1
  cplx2reim/1 -> dtc/1
  enable/1 -> Delay_ValidIn/1
  fft_data/1 -> cplx2reim/1
  delayMatch23/1 -> Out1/1
  Delay_ValidIn/1 -> invert_reset/1, DelayValidOut/1
  QuadrantMapper/2(yout) -> Iteration/2(yin)
  QuadrantMapper/1(xout) -> Iteration/1(xin)
  delayMatch1/1 -> QuadrantMapper/2(yin)
  delayMatch/1 -> QuadrantMapper/1(xin)
  delayMatch22/1 -> CSD Gain Factor/1
  delayMatch21/1 -> Iteration10/2(yin)
  delayMatch20/1 -> Iteration10/1(xin)
  delayMatch19/1 -> Iteration9/2(yin)
  delayMatch18/1 -> Iteration9/1(xin)
  delayMatch17/1 -> Iteration8/2(yin)
  delayMatch16/1 -> Iteration8/1(xin)
  delayMatch15/1 -> Iteration7/2(yin)
  delayMatch14/1 -> Iteration7/1(xin)
  delayMatch13/1 -> Iteration6/2(yin)
  delayMatch12/1 -> Iteration6/1(xin)
  delayMatch11/1 -> Iteration5/2(yin)
  delayMatch10/1 -> Iteration5/1(xin)
  delayMatch9/1 -> Iteration4/2(yin)
  delayMatch8/1 -> Iteration4/1(xin)
  delayMatch7/1 -> Iteration3/2(yin)
  delayMatch6/1 -> Iteration3/1(xin)
  delayMatch5/1 -> Iteration2/2(yin)
  delayMatch4/1 -> Iteration2/1(xin)
  delayMatch3/1 -> Iteration1/2(yin)
  delayMatch2/1 -> Iteration1/1(xin)
  DelayValidOut/1 -> Out2/1

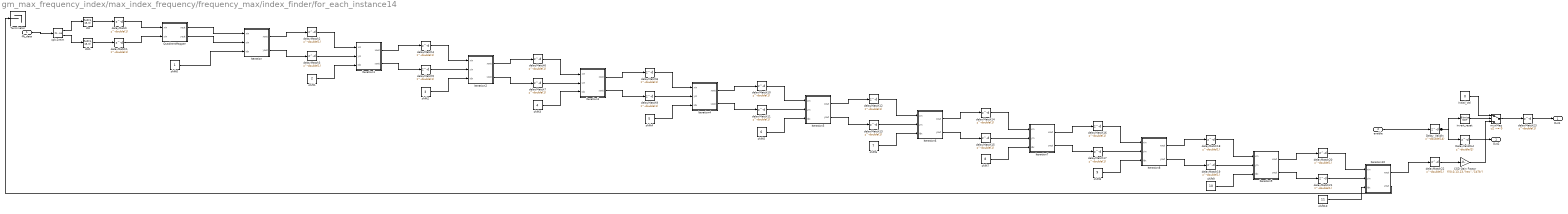
== system gm_max_frequency_index/max_index_frequency/frequency_max/index_finder/for_each_instance14 ==
  fft_data : Inport  OutDataTypeStr=fixdt(1, 12, 0)  PortDimensions=1  SampleTime=3.2e-05
      settings: SignalType=complex
  enable : Inport  Port=2  OutDataTypeStr=boolean  PortDimensions=1  SampleTime=3.2e-05
  CSD Gain Factor : Gain  Gain="fi(0,0,13,13,\"hex\",\"1b7b\")"  ParamDataTypeStr=fixdt(0, 13, 13)  OutDataTypeStr=fixdt(1, 13, 0)  SampleTime=3.2e-05
  DelayValidOut : Delay  DelayLength=double(1)  InitialCondition=0  SampleTime=3.2e-05
  Delay_ValidIn : Delay  DelayLength=double(14)  InitialCondition=0  SampleTime=3.2e-05
  Initial_Val : Constant  Value=0  OutDataTypeStr=fixdt(1, 13, 0)  SampleTime=3.2e-05
  Iteration : Subsystem
  Iteration1 : Subsystem
  Iteration10 : Subsystem
  Iteration2 : Subsystem
  Iteration3 : Subsystem
  Iteration4 : Subsystem
  Iteration5 : Subsystem
  Iteration6 : Subsystem
  Iteration7 : Subsystem
  Iteration8 : Subsystem
  Iteration9 : Subsystem
  QuadrantMapper : Subsystem
  Terminator : Terminator
  cplx2reim : ComplexToRealImag  SampleTime=3.2e-05
  delayMatch{,1..23} (24 alike) : Delay  DelayLength=double(1)  InitialCondition=0  SampleTime=3.2e-05
  dtc : DataTypeConversion  OutDataTypeStr=fixdt(1, 13, 0)  SampleTime=3.2e-05
  dtc1 : DataTypeConversion  OutDataTypeStr=fixdt(1, 13, 0)  SampleTime=3.2e-05
  invert_reset : simulink/Logic and Bit Operations/Bitwise Operator  logicop=NOT  UseBitMask=off  BitMask=double(0)  BitMaskRealWorld=Real World Value
  muxMag : Switch  Criteria=u2 ~= 0  Threshold=double(0)  OutDataTypeStr=fixdt(1, 13, 0)  SampleTime=3.2e-05
  shift0 : Constant  VectorParams1D=off  OutDataTypeStr=fixdt(0, 5, 0)  SampleTime=3.2e-05
  shift1 : Constant  Value=2  VectorParams1D=off  OutDataTypeStr=fixdt(0, 5, 0)  SampleTime=3.2e-05
  shift10 : Constant  Value=11  VectorParams1D=off  OutDataTypeStr=fixdt(0, 5, 0)  SampleTime=3.2e-05
  shift2 : Constant  Value=3  VectorParams1D=off  OutDataTypeStr=fixdt(0, 5, 0)  SampleTime=3.2e-05
  shift3 : Constant  Value=4  VectorParams1D=off  OutDataTypeStr=fixdt(0, 5, 0)  SampleTime=3.2e-05
  shift4 : Constant  Value=5  VectorParams1D=off  OutDataTypeStr=fixdt(0, 5, 0)  SampleTime=3.2e-05
  shift5 : Constant  Value=6  VectorParams1D=off  OutDataTypeStr=fixdt(0, 5, 0)  SampleTime=3.2e-05
  shift6 : Constant  Value=7  VectorParams1D=off  OutDataTypeStr=fixdt(0, 5, 0)  SampleTime=3.2e-05
  shift7 : Constant  Value=8  VectorParams1D=off  OutDataTypeStr=fixdt(0, 5, 0)  SampleTime=3.2e-05
  shift8 : Constant  Value=9  VectorParams1D=off  OutDataTypeStr=fixdt(0, 5, 0)  SampleTime=3.2e-05
  shift9 : Constant  Value=10  VectorParams1D=off  OutDataTypeStr=fixdt(0, 5, 0)  SampleTime=3.2e-05
  Out1 : Outport
  Out2 : Outport  Port=2  VectorParamsAs1DForOutWhenUnconnected=off
  wires:
  muxMag/1 -> delayMatch23/1
  invert_reset/1 -> muxMag/2
  CSD Gain Factor/1 -> muxMag/3
  Initial_Val/1 -> muxMag/1
  Iteration10/1(xout) -> delayMatch22/1
  shift10/1 -> Iteration10/3(idx)
  Iteration10/2(yout) -> Terminator/1
  Iteration9/2(yout) -> delayMatch21/1
  Iteration9/1(xout) -> delayMatch20/1
  shift9/1 -> Iteration9/3(idx)
  Iteration8/2(yout) -> delayMatch19/1
  Iteration8/1(xout) -> delayMatch18/1
  shift8/1 -> Iteration8/3(idx)
  Iteration7/2(yout) -> delayMatch17/1
  Iteration7/1(xout) -> delayMatch16/1
  shift7/1 -> Iteration7/3(idx)
  Iteration6/2(yout) -> delayMatch15/1
  Iteration6/1(xout) -> delayMatch14/1
  shift6/1 -> Iteration6/3(idx)
  Iteration5/2(yout) -> delayMatch13/1
  Iteration5/1(xout) -> delayMatch12/1
  shift5/1 -> Iteration5/3(idx)
  Iteration4/2(yout) -> delayMatch11/1
  Iteration4/1(xout) -> delayMatch10/1
  shift4/1 -> Iteration4/3(idx)
  Iteration3/2(yout) -> delayMatch9/1
  Iteration3/1(xout) -> delayMatch8/1
  shift3/1 -> Iteration3/3(idx)
  Iteration2/2(yout) -> delayMatch7/1
  Iteration2/1(xout) -> delayMatch6/1
  shift2/1 -> Iteration2/3(idx)
  Iteration1/2(yout) -> delayMatch5/1
  Iteration1/1(xout) -> delayMatch4/1
  shift1/1 -> Iteration1/3(idx)
  Iteration/2(yout) -> delayMatch3/1
  Iteration/1(xout) -> delayMatch2/1
  shift0/1 -> Iteration/3(idx)
  dtc1/1 -> delayMatch1/1
  dtc/1 -> delayMatch/1
  cplx2reim/2 -> dtc1/1
  cplx2reim/1 -> dtc/1
  enable/1 -> Delay_ValidIn/1
  fft_data/1 -> cplx2reim/1
  delayMatch23/1 -> Out1/1
  Delay_ValidIn/1 -> invert_reset/1, DelayValidOut/1
  QuadrantMapper/2(yout) -> Iteration/2(yin)
  QuadrantMapper/1(xout) -> Iteration/1(xin)
  delayMatch1/1 -> QuadrantMapper/2(yin)
  delayMatch/1 -> QuadrantMapper/1(xin)
  delayMatch22/1 -> CSD Gain Factor/1
  delayMatch21/1 -> Iteration10/2(yin)
  delayMatch20/1 -> Iteration10/1(xin)
  delayMatch19/1 -> Iteration9/2(yin)
  delayMatch18/1 -> Iteration9/1(xin)
  delayMatch17/1 -> Iteration8/2(yin)
  delayMatch16/1 -> Iteration8/1(xin)
  delayMatch15/1 -> Iteration7/2(yin)
  delayMatch14/1 -> Iteration7/1(xin)
  delayMatch13/1 -> Iteration6/2(yin)
  delayMatch12/1 -> Iteration6/1(xin)
  delayMatch11/1 -> Iteration5/2(yin)
  delayMatch10/1 -> Iteration5/1(xin)
  delayMatch9/1 -> Iteration4/2(yin)
  delayMatch8/1 -> Iteration4/1(xin)
  delayMatch7/1 -> Iteration3/2(yin)
  delayMatch6/1 -> Iteration3/1(xin)
  delayMatch5/1 -> Iteration2/2(yin)
  delayMatch4/1 -> Iteration2/1(xin)
  delayMatch3/1 -> Iteration1/2(yin)
  delayMatch2/1 -> Iteration1/1(xin)
  DelayValidOut/1 -> Out2/1
